simulink library "JointAngle2jointDynamics"  (R2016b)
settings: Solver=VariableStepAuto  StartTime=0.0  StopTime=10.0  RelTol=1e-3
libraries: simulink_extras x1
settings Model: Creator=Taeke  LastModifiedBy=Taeke

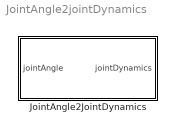
== system JointAngle2jointDynamics ==
  JointAngle2JointDynamics : Subsystem

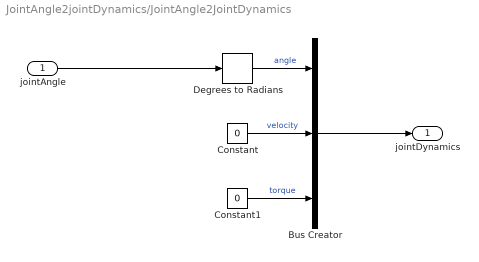
== system JointAngle2jointDynamics/JointAngle2JointDynamics ==
  jointAngle : Inport
  Bus Creator : BusCreator  Inputs=3  OutDataTypeStr=Bus: JointDynamics  NonVirtualBus=on
  Constant : Constant  Value=0
  Constant1 : Constant  Value=0
  Degrees to Radians : simulink_extras/Transformations/Degrees to Radians
  jointDynamics : Outport
  wires:
  Degrees to Radians/1 -> Bus Creator/1  "angle"
  Constant1/1 -> Bus Creator/3  "torque"
  jointAngle/1 -> Degrees to Radians/1
  Bus Creator/1 -> jointDynamics/1
  Constant/1 -> Bus Creator/2  "velocity"
